simulink model "CM745A_Sci30CfgAndUse"  (R2013b)
settings: Solver=ode45  StartTime=0.0  StopTime=10.0  RelTol=1e-3
libraries: simulink x12
(part 1 of 3)
settings Model: Creator=fz41t8  LastModifiedBy=fz41t8

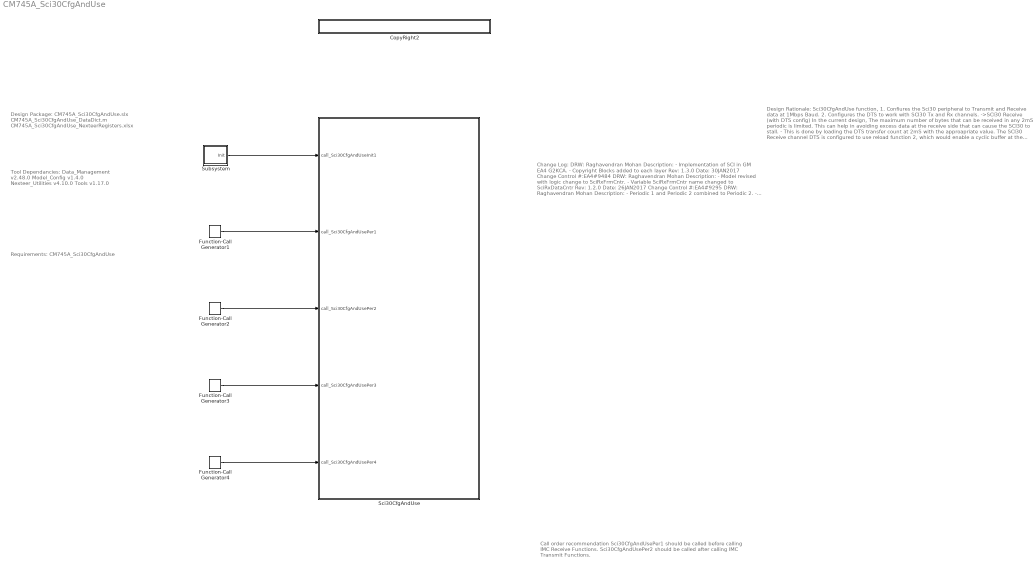
== system CM745A_Sci30CfgAndUse ==
  note: Call order recommendation
      |
      | Sci30CfgAndUsePer1 should be called before calling IMC Receive Functions.
      | Sci30CfgAndUsePer2 should be called after calling IMC Transmit Functions.
  note: Design Rationale:
      |
      | Sci30CfgAndUse function,
      | 1. Confiures the Sci30 peripheral to Transmit and Receive data at 1Mbps Baud.
      | 2. Configures the DTS to work with SCI30 Tx and Rx channels.
      |
      | ->SCI30 Receive (with DTS config)
      | In the current design, The maximum number of bytes that can be received in any
      | 2mS periodic is limited. This can help in avoiding excess data at the receive side
      | that can cause the SCI30 to stall.
      |  - This is done by loading the DTS transfer count at 2mS with the approapriate
      | value.
      | The SCI30 Receive channel DTS is configured to use reload function 2, which
      | would enable a cyclic buffer at the SCI30 receive.
      |  - This is done by configuring the address reload count. (Reload Function 2).
      |
      | ->SCI30 Transmit (with DTS config)
      | The amount of data to be sent out through the SCI30 Transmit channel is
      | loaded onto the DTS transfer count.(the number of DMA transfers equals
      | the amount of data sent out).
      | - This is done by reloading the DTS transfer count register with the actual
      |   amount of data.
      |
      | ->SCI30 Receive Channel Diagnostics
      | Sci30CfgAndUsePer2 function checks to see if the Sci receive channel has
      | received maximum amount of data and upon receiving maximum data it
      | checks for the overrun error, parity error or frame error and clears them if set.
      | This helps in preventing the SCI30 from stalling.
      |
      | Transmit - Channel master settings
      | SPID	2
      | PEID	1
      | UM		1
      |
      | Receive - Channel master settings
      | SPID	3
      | PEID	1
      | UM		1
      |
      | The DTS Channel Master settings need to be configured in SUPERVISOR Mode.
      |
      | Corruption of any of the registers would result in invalid data being sent to the other ECU.
      | And this would be the rationale behind why we dont need Protection for the SCI and DTS registers.
      | The SCI is not part of any protection, or PBG configuration.
      |
      |
      |
      | Sub-Function				rate (ms)
      |
      | Sci30CfgAndUsePer1			2			Required in all operating states
      | Sci30CfgAndUsePer2			2			Required in all operating states
      | Sci30CfgAndUsePer3			10			Required in all operating states
      | Sci30CfgAndUsePer4			100			Required in all operating states
  note: Design Package:
      |
      | CM745A_Sci30CfgAndUse.slx
      | CM745A_Sci30CfgAndUse_DataDict.m
      | CM745A_Sci30CfgAndUse_NexteerRegisters.xlsx
  note: Tool Dependancies:
      |
      | Data_Management v2.48.0
      | Model_Config v1.4.0
      | Nexteer_Utilities v4.10.0
      | Tools v1.17.0
  note: Change Log:
      |
      | DRW: Raghavendran Mohan
      | Description:
      | - Implementation of SCI in GM EA4 G2KCA.
      | - Copyright Blocks added to each layer
      |
      | Rev: 1.3.0
      | Date: 30JAN2017
      | Change Control #:EA4#9484
      | DRW: Raghavendran Mohan
      | Description:
      | - Model revised with logic change to SciRxFrmCntr.
      | - Variable SciRxFrmCntr name changed to SciRxDataCntr
      |
      | Rev: 1.2.0
      | Date: 26JAN2017
      | Change Control #:EA4#9295
      | DRW: Raghavendran Mohan
      | Description:
      | - Periodic 1 and Periodic 2 combined to Periodic 2.
      | - Periodic 5 changed to Periodic1.
      | - Name change for IMC dependent global constants.
      |
      | Rev: 1.1.0
      | Date: 11NOV2016
      | Change Control #:EA4#8302
      | DRW: Raghavendran Mohan
      | Description:
      | - Configured SCI30 to work with DTS
      | - Limited the number of messages to
      |   be received by SCI in any 2 mS
      |
      | Rev: 1.0.0
      | Date: 17OCT2016
      | Change Control #:EA4#7046
      | DRW: Raghavendran Mohan
      | Description:
      | - Initial Release
  note: Requirements:
      |
      | CM745A_Sci30CfgAndUse
  CopyRight2 : Subsystem  Description=|  mask(Copyright Information){none=on}
      | Copyright info block.                                               
      |                                                                     
      | Place copyright information at the top of every subsystem in design.
      mask prompts: none "No parameters"
      mask help: Place copyright information at the top of every subsystem in design.
      mask Display:
      | NxtrConf = 'Nexteer Confidential';
      | 
      | sys = bdroot; %handle for the current model ("system")
      | first = get_param(sys,'Created');
      | first = first(end-3:end);  %year is last four digits
      | 
      | last = get_param(sys,'LastModifiedDate');
      | if isempty(last)
      |     last = datestr(now,'yyyy');
      | else
      |     last = last(end-3:end);
      | end
      | 
      | if strcmp(first,last)
      |     fprintf('%s -- Copyright %s Nexteer',NxtrConf,first)
      | else
      |     fprintf('%s -- %s%s- %s Nexteer',NxtrConf,char(169),first,last)
      | end
  Function-Call Generator1 : simulink/Ports & Subsystems/Function-Call Generator  sample_time=0.002  numberOfIterations=1
      settings: AttributesFormatString=%<sample_time>
  Function-Call Generator2 : simulink/Ports & Subsystems/Function-Call Generator  sample_time=0.002  numberOfIterations=1
      settings: AttributesFormatString=%<sample_time>
  Function-Call Generator3 : simulink/Ports & Subsystems/Function-Call Generator  sample_time=0.01  numberOfIterations=1
      settings: AttributesFormatString=%<sample_time>
  Function-Call Generator4 : simulink/Ports & Subsystems/Function-Call Generator  sample_time=0.1  numberOfIterations=1
      settings: AttributesFormatString=%<sample_time>
  Sci30CfgAndUse : Subsystem
  Subsystem : Subsystem
  wires:
  Function-Call Generator1/1 -> Sci30CfgAndUse/2(call_Sci30CfgAndUsePer1)
  Function-Call Generator2/1 -> Sci30CfgAndUse/3(call_Sci30CfgAndUsePer2)
  Function-Call Generator3/1 -> Sci30CfgAndUse/4(call_Sci30CfgAndUsePer3)
  Function-Call Generator4/1 -> Sci30CfgAndUse/5(call_Sci30CfgAndUsePer4)
  Subsystem/1(Init) -> Sci30CfgAndUse/1(call_Sci30CfgAndUseInit1)

== system CM745A_Sci30CfgAndUse/CopyRight2 ==

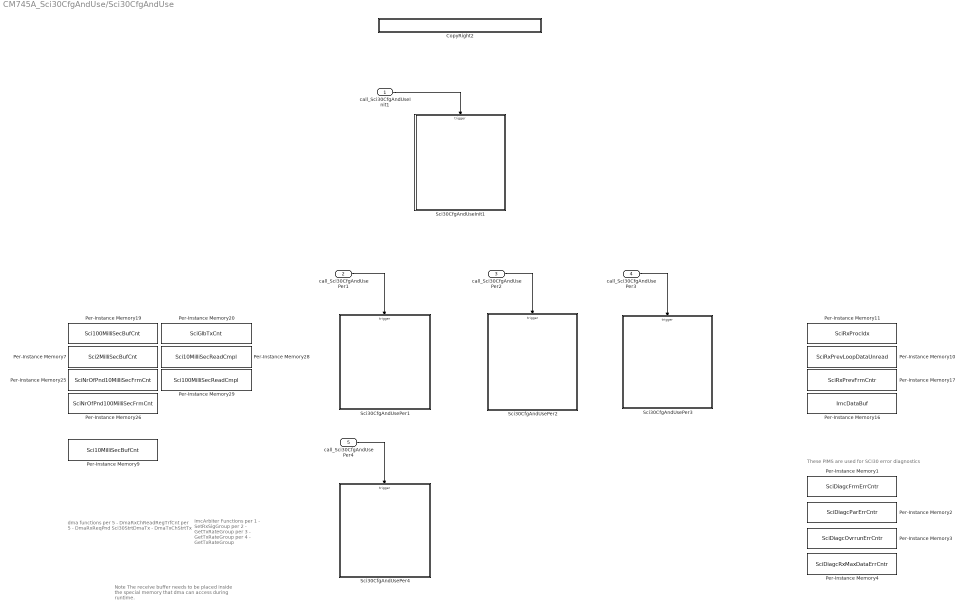
== system CM745A_Sci30CfgAndUse/Sci30CfgAndUse ==
  note: These PIMS are used for SCI30 error diagnostics
  note: Note
      |
      | The receive buffer needs to be placed
      | inside the special memory that dma can access
      |  during runtime.
  note: ImcArbiter Functions
      |
      | per 1 - SetRxSigGroup
      | per 2 - GetTxRateGroup
      | per 3 - GetTxRateGroup
      | per 4 - GetTxRateGroup
  note: dma functions
      |
      | per 5 - 				DmaRxChReadRegTrfCnt
      | per 5 - 				DmaRxReqPnd
      | Sci30StrtDmaTx - 	DmaTxChStrtTx
  call_Sci30CfgAndUseInit1 : Inport
  call_Sci30CfgAndUsePer1 : Inport  Port=2
  call_Sci30CfgAndUsePer2 : Inport  Port=3
  call_Sci30CfgAndUsePer3 : Inport  Port=4
  call_Sci30CfgAndUsePer4 : Inport  Port=5
  CopyRight2 : Subsystem  Description=|  mask(Copyright Information){none=on}
      | Copyright info block.                                               
      |                                                                     
      | Place copyright information at the top of every subsystem in design.
      mask prompts: none "No parameters"
      mask help: Place copyright information at the top of every subsystem in design.
      mask Display:
      | NxtrConf = 'Nexteer Confidential';
      | 
      | sys = bdroot; %handle for the current model ("system")
      | first = get_param(sys,'Created');
      | first = first(end-3:end);  %year is last four digits
      | 
      | last = get_param(sys,'LastModifiedDate');
      | if isempty(last)
      |     last = datestr(now,'yyyy');
      | else
      |     last = last(end-3:end);
      | end
      | 
      | if strcmp(first,last)
      |     fprintf('%s -- Copyright %s Nexteer',NxtrConf,first)
      | else
      |     fprintf('%s -- %s%s- %s Nexteer',NxtrConf,char(169),first,last)
      | end
  Per-Instance Memory1 : DataStoreMemory  RequirementInfo={} %GIDa_b3b57849_cbb3_4377_a3cb_912e17b0b2a0  DataStoreName=SciDiagcFrmErrCntr  OutDataTypeStr=uint32  StateMustResolveToSignalObject=on
  Per-Instance Memory10 : DataStoreMemory  RequirementInfo={} %GIDa_4ed7bc09_7e9a_458d_afd1_2a330d829650  DataStoreName=SciRxPrevLoopDataUnread  StateMustResolveToSignalObject=on
  Per-Instance Memory11 : DataStoreMemory  RequirementInfo={} %GIDa_3ccbf926_e816_4ba1_aa33_6f8a7244583b  DataStoreName=SciRxProcIdx  StateMustResolveToSignalObject=on
  Per-Instance Memory16 : DataStoreMemory  RequirementInfo={} %GIDa_a4699ec3_7b23_4e85_92c1_3b8b276d6679  DataStoreName=ImcDataBuf  InitialValue=[0,0,0,0,0,0,0,0]  OutDataTypeStr=uint8
  Per-Instance Memory17 : DataStoreMemory  RequirementInfo={} %GIDa_b61881d6_4c07_453b_890e_34f27dc90187  DataStoreName=SciRxPrevFrmCntr  StateMustResolveToSignalObject=on
  Per-Instance Memory19 : DataStoreMemory  RequirementInfo={} %GIDa_ab8726e9_5ac4_4e9c_b3bf_e5d79526c9cb  DataStoreName=Sci100MilliSecBufCnt  InitialValue=[]  VectorParams1D=off  StateMustResolveToSignalObject=on
  Per-Instance Memory2 : DataStoreMemory  RequirementInfo={} %GIDa_88ddc365_cba9_41ff_9af8_4f3bc4bcdd94  DataStoreName=SciDiagcParErrCntr  OutDataTypeStr=uint32  StateMustResolveToSignalObject=on
  Per-Instance Memory20 : DataStoreMemory  RequirementInfo={} %GIDa_d7519dc7_a6fd_4090_8a65_d6acf3c90b4e  DataStoreName=SciGlbTxCnt  OutDataTypeStr=uint8
  Per-Instance Memory25 : DataStoreMemory  RequirementInfo={} %GIDa_d42e51a1_a818_4595_ab2d_fbf8ed86b046  DataStoreName=SciNrOfPnd10MilliSecFrmCnt  OutDataTypeStr=uint8  StateMustResolveToSignalObject=on
  Per-Instance Memory26 : DataStoreMemory  RequirementInfo={} %GIDa_f5e07739_10f3_40b7_aa65_e2f998123e89  DataStoreName=SciNrOfPnd100MilliSecFrmCnt  OutDataTypeStr=uint8  StateMustResolveToSignalObject=on
  Per-Instance Memory28 : DataStoreMemory  RequirementInfo={} %GIDa_48b46abc_e5dd_4b66_8fa5_e2298010fa14  DataStoreName=Sci10MilliSecReadCmpl  OutDataTypeStr=boolean  StateMustResolveToSignalObject=on
  Per-Instance Memory29 : DataStoreMemory  RequirementInfo={} %GIDa_dd6879f0_97cd_4846_96b6_db1da32b280f  DataStoreName=Sci100MilliSecReadCmpl  OutDataTypeStr=boolean  StateMustResolveToSignalObject=on
  Per-Instance Memory3 : DataStoreMemory  RequirementInfo={} %GIDa_7153fc19_d7c8_405e_b0c8_79396bfd99b1  DataStoreName=SciDiagcOvrrunErrCntr  OutDataTypeStr=uint32  StateMustResolveToSignalObject=on
  Per-Instance Memory4 : DataStoreMemory  RequirementInfo={} %GIDa_3839a9f4_ebd7_4d8c_aa5f_02934402c7a8  DataStoreName=SciDiagcRxMaxDataErrCntr  OutDataTypeStr=uint32  StateMustResolveToSignalObject=on
  Per-Instance Memory7 : DataStoreMemory  RequirementInfo={} %GIDa_9668f34c_3dff_4881_9619_19e89a11e5d7  DataStoreName=Sci2MilliSecBufCnt  InitialValue=[]  OutDataTypeStr=uint8  StateMustResolveToSignalObject=on
  Per-Instance Memory9 : DataStoreMemory  RequirementInfo={} %GIDa_355f0922_cfd3_4bc4_b51e_9084d08cfe53  DataStoreName=Sci10MilliSecBufCnt  InitialValue=[]  OutDataTypeStr=uint8  StateMustResolveToSignalObject=on
  Sci30CfgAndUseInit1 : Subsystem  TreatAsAtomicUnit=on
  Sci30CfgAndUsePer1 : Subsystem  RequirementInfo={'linktype_rmi_doors' '00011b59 (/ESG Group/FDD Module Requirements/EA4 Specific/CM745A_Sci30CfgAndUse)' '#CM745A_28' 'true' 'REQ: CM745A_28' '' } %GIDa_bf038dd7_1ab4_4b18_b135_ed2bcc78b1b0  TreatAsAtomicUnit=on
  Sci30CfgAndUsePer2 : Subsystem  RequirementInfo={'linktype_rmi_doors' '00011b59 (/ESG Group/FDD Module Requirements/EA4 Specific/CM745A_Sci30CfgAndUse)' '#CM745A_25' 'true' 'REQ: CM745A_25' '' } %GIDa_256e35fd_67e5_4b63_bd20_7618d4918bb6  TreatAsAtomicUnit=on
  Sci30CfgAndUsePer3 : Subsystem  RequirementInfo={'linktype_rmi_doors' '00011b59 (/ESG Group/FDD Module Requirements/EA4 Specific/CM745A_Sci30CfgAndUse)' '#CM745A_26' 'true' 'REQ: CM745A_26' '' } %GIDa_9e620a39_8a29_406c_9071_7abfd40cb07e  TreatAsAtomicUnit=on
  Sci30CfgAndUsePer4 : Subsystem  RequirementInfo={'linktype_rmi_doors' '00011b59 (/ESG Group/FDD Module Requirements/EA4 Specific/CM745A_Sci30CfgAndUse)' '#CM745A_27' 'true' 'REQ: CM745A_27' '' } %GIDa_e30a56bb_70ac_43bc_bb33_116577e74951  TreatAsAtomicUnit=on
  wires:
  call_Sci30CfgAndUseInit1/1 -> Sci30CfgAndUseInit1/Trigger
  call_Sci30CfgAndUsePer1/1 -> Sci30CfgAndUsePer1/Trigger
  call_Sci30CfgAndUsePer2/1 -> Sci30CfgAndUsePer2/Trigger
  call_Sci30CfgAndUsePer3/1 -> Sci30CfgAndUsePer3/Trigger
  call_Sci30CfgAndUsePer4/1 -> Sci30CfgAndUsePer4/Trigger

== system CM745A_Sci30CfgAndUse/Subsystem ==
  CopyRight2 : Subsystem  Description=|  mask(Copyright Information){none=on}
      | Copyright info block.                                               
      |                                                                     
      | Place copyright information at the top of every subsystem in design.
      mask prompts: none "No parameters"
      mask help: Place copyright information at the top of every subsystem in design.
      mask Display:
      | NxtrConf = 'Nexteer Confidential';
      | 
      | sys = bdroot; %handle for the current model ("system")
      | first = get_param(sys,'Created');
      | first = first(end-3:end);  %year is last four digits
      | 
      | last = get_param(sys,'LastModifiedDate');
      | if isempty(last)
      |     last = datestr(now,'yyyy');
      | else
      |     last = last(end-3:end);
      | end
      | 
      | if strcmp(first,last)
      |     fprintf('%s -- Copyright %s Nexteer',NxtrConf,first)
      | else
      |     fprintf('%s -- %s%s- %s Nexteer',NxtrConf,char(169),first,last)
      | end
  Enabled Subsystem : Subsystem  TreatAsAtomicUnit=on
  Step : Step  Before=1  After=0  SampleTime=0
  Init : Outport
  wires:
  Enabled Subsystem/1(Init) -> Init/1
  Step/1 -> Enabled Subsystem/Enable

== system CM745A_Sci30CfgAndUse/Sci30CfgAndUse/CopyRight2 ==

== system CM745A_Sci30CfgAndUse/Sci30CfgAndUse/Sci30CfgAndUseInit1 ==
  note: This Function initializes the SCI30 Tx and Rx channels to communicate at 1Mbps Baud Rate.
      | This Function configures the DTS to work with SCI30 Tx(DTS 88) and Rx(DTS 87).
  note: DMA-DTS Register Configuration
  note: Configure SCI30 peripheral using sheet NexteerSCI30Registers inside CM745A_Sci30CfgAndUse_NexteerRegisters.xlsx
  note: Please find SCI30 DTS register configurations in SCI30CfgAndUseDTS.xlsx
      |
      | PSEUDO CODE
      |
      |
      | DTS CHANNEL 88 SCI30 TRANSMIT CONFIGURATION
      |
      | DMASSDTFSL088 = 0;
      | DMASSDTSA088 = (uint32)&SciGlbTxBuf[0];
      | DMASSDTDA088 = (uint32)&SCI30TDR;
      | DMASSDTTC088 = 0;
      | DMASSDTTCT088 = 256;
      |
      | DMASSDTFSC088 = 1;
      | DMASSDTFSL088 = 1;
      |
      |
      |
      | DTS CHANNEL 87 SCI30 RECEIVE CONFIGURATION
      |
      | DMASSDTFSL087 = 0;
      | DMASSDTSA087 = (uint32)&SCI30RDR;
      | DMASSDTDA087 = (uint32)&SciGlbRxBuf[0];
      | DMASSDTTC087 = 8388736;
      | DMASSDTTCT087 = 6208;
      |
      | DMASSDTRSA087 = (uint32)&SCI30RDR;
      | DMASSDTRDA087 = (uint32)&SciGlbRxBuf[0];
      | DMASSDTRTC087 |= 8388608;
      |
      | DMASSDTFSC087 = 1;
      | DMASSDTFSL087 = 1;
  note: Configure DMA DTS channel 87 and 88 using sheet NexteerDTSRegisters inside CM745A_Sci30CfgAndUse_NexteerRegisters.xlsx
  function : TriggerPort  TriggerType=function-call
  CopyRight2 : Subsystem  Description=|  mask(Copyright Information){none=on}
      | Copyright info block.                                               
      |                                                                     
      | Place copyright information at the top of every subsystem in design.
      mask prompts: none "No parameters"
      mask help: Place copyright information at the top of every subsystem in design.
      mask Display:
      | NxtrConf = 'Nexteer Confidential';
      | 
      | sys = bdroot; %handle for the current model ("system")
      | first = get_param(sys,'Created');
      | first = first(end-3:end);  %year is last four digits
      | 
      | last = get_param(sys,'LastModifiedDate');
      | if isempty(last)
      |     last = datestr(now,'yyyy');
      | else
      |     last = last(end-3:end);
      | end
      | 
      | if strcmp(first,last)
      |     fprintf('%s -- Copyright %s Nexteer',NxtrConf,first)
      | else
      |     fprintf('%s -- %s%s- %s Nexteer',NxtrConf,char(169),first,last)
      | end

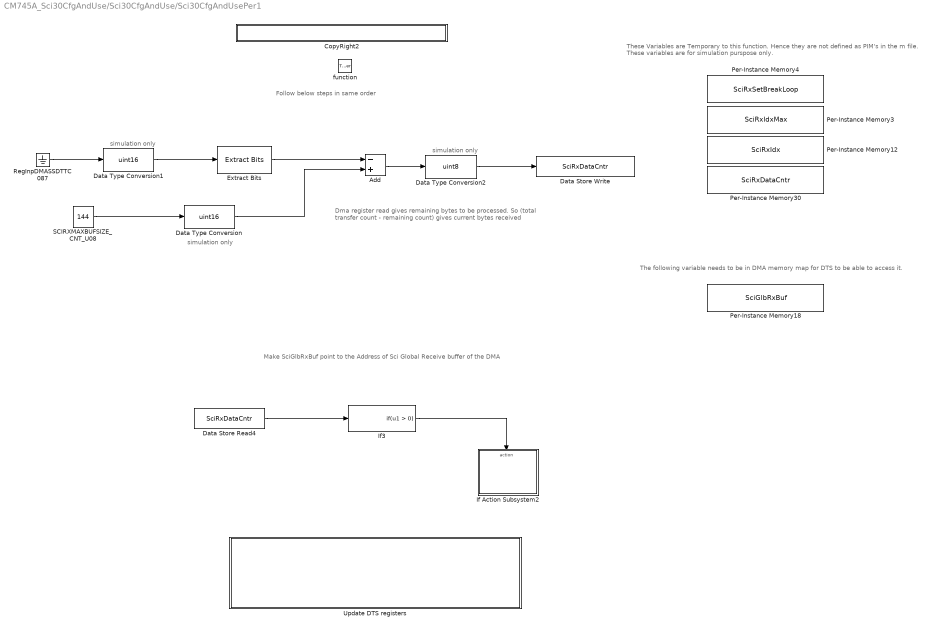
== system CM745A_Sci30CfgAndUse/Sci30CfgAndUse/Sci30CfgAndUsePer1 ==
  note: simulation only
  note: Dma register read gives remaining bytes to be processed.
      | So (total transfer count - remaining count) gives current bytes received
  note: Make SciGlbRxBuf point to the Address of Sci Global Receive buffer of the DMA
  note: Follow below steps in same order
  note: These Variables are Temporary to this function. Hence they are not defined as PIM's in the m file.
      | These variables are for simulation purspose only.
  note: simulation only
  note: simulation only
  note: The following variable needs to be in DMA memory map for DTS to be able to access it.
  function : TriggerPort  TriggerType=function-call
  Add : Sum  Inputs=-+
  CopyRight2 : Subsystem  Description=|  mask(Copyright Information){none=on}
      | Copyright info block.                                               
      |                                                                     
      | Place copyright information at the top of every subsystem in design.
      mask prompts: none "No parameters"
      mask help: Place copyright information at the top of every subsystem in design.
      mask Display:
      | NxtrConf = 'Nexteer Confidential';
      | 
      | sys = bdroot; %handle for the current model ("system")
      | first = get_param(sys,'Created');
      | first = first(end-3:end);  %year is last four digits
      | 
      | last = get_param(sys,'LastModifiedDate');
      | if isempty(last)
      |     last = datestr(now,'yyyy');
      | else
      |     last = last(end-3:end);
      | end
      | 
      | if strcmp(first,last)
      |     fprintf('%s -- Copyright %s Nexteer',NxtrConf,first)
      | else
      |     fprintf('%s -- %s%s- %s Nexteer',NxtrConf,char(169),first,last)
      | end
  Data Store Read4 : DataStoreRead  DataStoreName=SciRxDataCntr
  Data Store Write : DataStoreWrite  DataStoreName=SciRxDataCntr
  Data Type Conversion : DataTypeConversion  OutDataTypeStr=uint16
  Data Type Conversion1 : DataTypeConversion  OutDataTypeStr=uint16
  Data Type Conversion2 : DataTypeConversion  OutDataTypeStr=uint8
  Extract Bits : simulink/Logic and Bit Operations/Extract Bits  bitsToExtract=Range of bits  numBits=8  bitIdxRange=[0 15]  outScalingMode=Preserve fixed-point scaling
  If Action Subsystem2 : Subsystem  TreatAsAtomicUnit=on
  If3 : If  ShowElse=off
      settings: AttributesFormatString=%<IfExpression>
  Per-Instance Memory12 : DataStoreMemory  RequirementInfo={} %GIDa_10aec818_c7eb_44be_9468_3f861d56c791  DataStoreName=SciRxIdx  OutDataTypeStr=uint8
  Per-Instance Memory18 : DataStoreMemory  RequirementInfo={} %GIDa_9eb3493f_f4d3_4ae6_8599_8ce3936fda0e  DataStoreName=SciGlbRxBuf  InitialValue=[0,0,0,0,0,0,0,0]  OutDataTypeStr=uint8
  Per-Instance Memory3 : DataStoreMemory  RequirementInfo={} %GIDa_0f1d5dec_99dd_48b3_81e2_7cc92f58afeb  DataStoreName=SciRxIdxMax  OutDataTypeStr=uint8
  Per-Instance Memory30 : DataStoreMemory  RequirementInfo={} %GIDa_67fcd88a_9e09_4a74_a9c0_611da1fab4fa  DataStoreName=SciRxDataCntr
  Per-Instance Memory4 : DataStoreMemory  RequirementInfo={} %GIDa_846dd6da_f32a_4fb1_951f_9840ad07db99  DataStoreName=SciRxSetBreakLoop  OutDataTypeStr=boolean
  RegInpDMASSDTTC087 : Ground
  SCIRXMAXBUFSIZE_CNT_U08 : Constant  Value=144  OutDataTypeStr=uint8
  Update DTS registers : Subsystem
  wires:
  Data Store Read4/1 -> If3/1
  If3/1 -> If Action Subsystem2/Action
  Extract Bits/1 -> Add/1
  Data Type Conversion1/1 -> Extract Bits/1
  RegInpDMASSDTTC087/1 -> Data Type Conversion1/1
  SCIRXMAXBUFSIZE_CNT_U08/1 -> Data Type Conversion/1
  Data Type Conversion/1 -> Add/2
  Data Type Conversion2/1 -> Data Store Write/1
  Add/1 -> Data Type Conversion2/1

== system CM745A_Sci30CfgAndUse/Sci30CfgAndUse/Sci30CfgAndUsePer2 ==
  note: This Data needs to be put in exclusive
      | memory, that has read/write protection.
      | (To prevent Read Write Collision)
  note: Conditional Compile (Based on IMC Arbitration of 2 Millisec Rate Group !=0)
  note: Follow below steps in same order
  note: This Data needs to be put in exclusive
      | memory, that has read/write protection.
      | (To prevent Read Write Collision)
  function : TriggerPort  TriggerType=function-call
  CopyRight2 : Subsystem  Description=|  mask(Copyright Information){none=on}
      | Copyright info block.                                               
      |                                                                     
      | Place copyright information at the top of every subsystem in design.
      mask prompts: none "No parameters"
      mask help: Place copyright information at the top of every subsystem in design.
      mask Display:
      | NxtrConf = 'Nexteer Confidential';
      | 
      | sys = bdroot; %handle for the current model ("system")
      | first = get_param(sys,'Created');
      | first = first(end-3:end);  %year is last four digits
      | 
      | last = get_param(sys,'LastModifiedDate');
      | if isempty(last)
      |     last = datestr(now,'yyyy');
      | else
      |     last = last(end-3:end);
      | end
      | 
      | if strcmp(first,last)
      |     fprintf('%s -- Copyright %s Nexteer',NxtrConf,first)
      | else
      |     fprintf('%s -- %s%s- %s Nexteer',NxtrConf,char(169),first,last)
      | end
  Data Store Read1 : DataStoreRead  DataStoreName=Sci2MilliSecBufCnt
  Data Store Write1 : DataStoreWrite  DataStoreName=Sci2MilliSecReadCmpl
  GetTxRateGroup : Subsystem
  IMCARBN_NROF2MILLISECRATEGROUP_CNT_U08 : Constant  Value=0  OutDataTypeStr=uint8
  IMCARBN_RATEGROUPID2MILLISEC_CNT_U08 : Constant  Value=0  OutDataTypeStr=uint8
  Per-Instance Memory27 : DataStoreMemory  RequirementInfo={} %GIDa_fa2153ee_75ad_4194_bafc_e32e8d6d4301  DataStoreName=Sci2MilliSecReadCmpl  OutDataTypeStr=boolean
  Sci30Transmit : Subsystem  RequirementInfo={'linktype_rmi_doors' '00011b59 (/ESG Group/FDD Module Requirements/EA4 Specific/CM745A_Sci30CfgAndUse)' '#CM745A_24' 'true' 'REQ: CM745A_24' '' } %GIDa_898b519a_4f36_4d71_a508_ee16e2031590  TreatAsAtomicUnit=on
  Terminator : Terminator
  wires:
  IMCARBN_NROF2MILLISECRATEGROUP_CNT_U08/1 -> Terminator/1
  GetTxRateGroup/1(Sci2MilliSecReadCmplCnt) -> Data Store Write1/1
  Data Store Read1/1 -> GetTxRateGroup/2(Sci2MilliSecBufCnt)
  IMCARBN_RATEGROUPID2MILLISEC_CNT_U08/1 -> GetTxRateGroup/1(IMCARBN_RATEGROUPID2MILLISEC)

== system CM745A_Sci30CfgAndUse/Sci30CfgAndUse/Sci30CfgAndUsePer3 ==
  note: Conditional Compile (Based on IMC Arbitration of 2 Millisec Rate Group !=0)
  note: Follow below steps in same order
  note: This Data needs to be put in exclusive
      | memory, that has read/write protection.
      | (To prevent Read Write Collision)
  note: This Data needs to be put in exclusive
      | memory, that has read/write protection.
      | (To prevent Read Write Collision)
  note: This Data needs to be put in exclusive
      | memory, that has read/write protection.
      | (To prevent Read Write Collision)
  function : TriggerPort  TriggerType=function-call
  CopyRight2 : Subsystem  Description=|  mask(Copyright Information){none=on}
      | Copyright info block.                                               
      |                                                                     
      | Place copyright information at the top of every subsystem in design.
      mask prompts: none "No parameters"
      mask help: Place copyright information at the top of every subsystem in design.
      mask Display:
      | NxtrConf = 'Nexteer Confidential';
      | 
      | sys = bdroot; %handle for the current model ("system")
      | first = get_param(sys,'Created');
      | first = first(end-3:end);  %year is last four digits
      | 
      | last = get_param(sys,'LastModifiedDate');
      | if isempty(last)
      |     last = datestr(now,'yyyy');
      | else
      |     last = last(end-3:end);
      | end
      | 
      | if strcmp(first,last)
      |     fprintf('%s -- Copyright %s Nexteer',NxtrConf,first)
      | else
      |     fprintf('%s -- %s%s- %s Nexteer',NxtrConf,char(169),first,last)
      | end
  Data Store Read1 : DataStoreRead  DataStoreName=Sci10MilliSecBufCnt
  Data Store Write : DataStoreWrite  DataStoreName=SciNrOfPnd10MilliSecFrmCnt
  Data Store Write1 : DataStoreWrite  DataStoreName=Sci10MilliSecReadCmpl
  GetTxRateGroup : Subsystem
  IMCARBN_NROF10MILLISECRATEGROUP_CNT_U08 : Constant  Value=0  OutDataTypeStr=uint8
  IMCARBN_RATEGROUPID10MILLISEC_CNT_U08 : Constant  Value=0  OutDataTypeStr=uint8
  wires:
  IMCARBN_NROF10MILLISECRATEGROUP_CNT_U08/1 -> Data Store Write/1
  GetTxRateGroup/1(Sci10MilliSecReadCmplCnt) -> Data Store Write1/1
  Data Store Read1/1 -> GetTxRateGroup/2(Sci10MilliSecBufCnt)
  IMCARBN_RATEGROUPID10MILLISEC_CNT_U08/1 -> GetTxRateGroup/1(IMCARBN_RATEGROUPID10MILLISEC)

== system CM745A_Sci30CfgAndUse/Sci30CfgAndUse/Sci30CfgAndUsePer4 ==
  note: Follow below steps in same order
  note: Conditional Compile (Based on IMC Arbitration of 2 Millisec Rate Group !=0)
  note: This Data needs to be put in exclusive
      | memory, that has read/write protection.
      | (To prevent Read Write Collision)
  note: This Data needs to be put in exclusive
      | memory, that has read/write protection.
      | (To prevent Read Write Collision)
  note: This Data needs to be put in exclusive
      | memory, that has read/write protection.
      | (To prevent Read Write Collision)
  function : TriggerPort  TriggerType=function-call
  CopyRight2 : Subsystem  Description=|  mask(Copyright Information){none=on}
      | Copyright info block.                                               
      |                                                                     
      | Place copyright information at the top of every subsystem in design.
      mask prompts: none "No parameters"
      mask help: Place copyright information at the top of every subsystem in design.
      mask Display:
      | NxtrConf = 'Nexteer Confidential';
      | 
      | sys = bdroot; %handle for the current model ("system")
      | first = get_param(sys,'Created');
      | first = first(end-3:end);  %year is last four digits
      | 
      | last = get_param(sys,'LastModifiedDate');
      | if isempty(last)
      |     last = datestr(now,'yyyy');
      | else
      |     last = last(end-3:end);
      | end
      | 
      | if strcmp(first,last)
      |     fprintf('%s -- Copyright %s Nexteer',NxtrConf,first)
      | else
      |     fprintf('%s -- %s%s- %s Nexteer',NxtrConf,char(169),first,last)
      | end
  Data Store Read1 : DataStoreRead  DataStoreName=Sci100MilliSecBufCnt
  Data Store Write : DataStoreWrite  DataStoreName=SciNrOfPnd100MilliSecFrmCnt
  Data Store Write1 : DataStoreWrite  DataStoreName=Sci100MilliSecReadCmpl
  GetTxRateGroup : Subsystem
  IMCARBN_NROF100MILLISECRATEGROUP_CNT_U08 : Constant  OutDataTypeStr=uint8
  IMCARBN_RATEGROUPID100MILLISEC_CNT_U08 : Constant  OutDataTypeStr=uint8
  wires:
  IMCARBN_NROF100MILLISECRATEGROUP_CNT_U08/1 -> Data Store Write/1
  GetTxRateGroup/1(Sci100MilliSecReadCmplCnt) -> Data Store Write1/1
  Data Store Read1/1 -> GetTxRateGroup/2(Sci100MilliSecBufCnt)
  IMCARBN_RATEGROUPID100MILLISEC_CNT_U08/1 -> GetTxRateGroup/1(IMCARBN_RATEGROUPID100MILLISEC)

== system CM745A_Sci30CfgAndUse/Subsystem/CopyRight2 ==

== system CM745A_Sci30CfgAndUse/Subsystem/Enabled Subsystem ==
  Enable : EnablePort
  CopyRight2 : Subsystem  Description=|  mask(Copyright Information){none=on}
      | Copyright info block.                                               
      |                                                                     
      | Place copyright information at the top of every subsystem in design.
      mask prompts: none "No parameters"
      mask help: Place copyright information at the top of every subsystem in design.
      mask Display:
      | NxtrConf = 'Nexteer Confidential';
      | 
      | sys = bdroot; %handle for the current model ("system")
      | first = get_param(sys,'Created');
      | first = first(end-3:end);  %year is last four digits
      | 
      | last = get_param(sys,'LastModifiedDate');
      | if isempty(last)
      |     last = datestr(now,'yyyy');
      | else
      |     last = last(end-3:end);
      | end
      | 
      | if strcmp(first,last)
      |     fprintf('%s -- Copyright %s Nexteer',NxtrConf,first)
      | else
      |     fprintf('%s -- %s%s- %s Nexteer',NxtrConf,char(169),first,last)
      | end
  Function Call Trigger : simulink/Ports & Subsystems/Function-Call Generator  RequirementInfo="{'linktype_rmi_doors' '000089e3 (/E-STEER_New/System Specification Documents/Core Specs/Subsystem Specs/System Functions FDD/SF-46  Gross Cross Check)' '#211' 'true' 'REQ: SF046A_211' '' ; 'linktype_rmi_doors' '000089e3 (/E-STEER_New/System Specification Documents/Core Specs/Subsystem Specs/System Functions FDD/SF-46  Gross Cross Check)' '#182' 'true' 'REQ: SF046A_182' '' } %GIDa_cf5bacff_48a9_4312_b446_700ab36e3d94"  sample_time=0.002  numberOfIterations=1
      settings: AttributesFormatString=%<sample_time>
  Init : Outport
  wires:
  Function Call Trigger/1 -> Init/1

== system CM745A_Sci30CfgAndUse/Sci30CfgAndUse/Sci30CfgAndUseInit1/CopyRight2 ==

== system CM745A_Sci30CfgAndUse/Sci30CfgAndUse/Sci30CfgAndUsePer1/CopyRight2 ==

== system CM745A_Sci30CfgAndUse/Sci30CfgAndUse/Sci30CfgAndUsePer1/If Action Subsystem2 ==
  note: Follow below steps in same order
  Action Port : ActionPort  ActionType=then
  Add : Sum
  Constant : Constant  Value=0  OutDataTypeStr=boolean
  Constant1 : Constant  Value=0  OutDataTypeStr=uint8
  Constant2 : Constant  Value=0  OutDataTypeStr=uint8
  CopyRight2 : Subsystem  Description=|  mask(Copyright Information){none=on}
      | Copyright info block.                                               
      |                                                                     
      | Place copyright information at the top of every subsystem in design.
      mask prompts: none "No parameters"
      mask help: Place copyright information at the top of every subsystem in design.
      mask Display:
      | NxtrConf = 'Nexteer Confidential';
      | 
      | sys = bdroot; %handle for the current model ("system")
      | first = get_param(sys,'Created');
      | first = first(end-3:end);  %year is last four digits
      | 
      | last = get_param(sys,'LastModifiedDate');
      | if isempty(last)
      |     last = datestr(now,'yyyy');
      | else
      |     last = last(end-3:end);
      | end
      | 
      | if strcmp(first,last)
      |     fprintf('%s -- Copyright %s Nexteer',NxtrConf,first)
      | else
      |     fprintf('%s -- %s%s- %s Nexteer',NxtrConf,char(169),first,last)
      | end
  Data Store Read1 : DataStoreRead  DataStoreName=SciRxDataCntr
  Data Store Read3 : DataStoreRead  DataStoreName=SciRxPrevLoopDataUnread
  Data Store Read4 : DataStoreRead  DataStoreName=SciRxDataCntr
  Data Store Write : DataStoreWrite  DataStoreName=SciRxIdx
  Data Store Write1 : DataStoreWrite  DataStoreName=SciRxPrevLoopDataUnread
  Data Store Write2 : DataStoreWrite  DataStoreName=SciRxIdxMax
  Data Store Write3 : DataStoreWrite  DataStoreName=SciRxPrevFrmCntr
  While Iterator Subsystem : Subsystem  RequirementInfo={'linktype_rmi_doors' '00011b59 (/ESG Group/FDD Module Requirements/EA4 Specific/CM745A_Sci30CfgAndUse)' '#CM745A_35' 'true' 'REQ: CM745A_35' '' } %GIDa_a7febead_a2f3_48b5_a7e9_dbc4923b1949  TreatAsAtomicUnit=on
  wires:
  Constant/1 -> While Iterator Subsystem/1(IC)
  Data Store Read1/1 -> Data Store Write3/1
  Constant1/1 -> Data Store Write/1
  Constant2/1 -> Data Store Write1/1
  Data Store Read3/1 -> Add/2
  Add/1 -> Data Store Write2/1
  Data Store Read4/1 -> Add/1

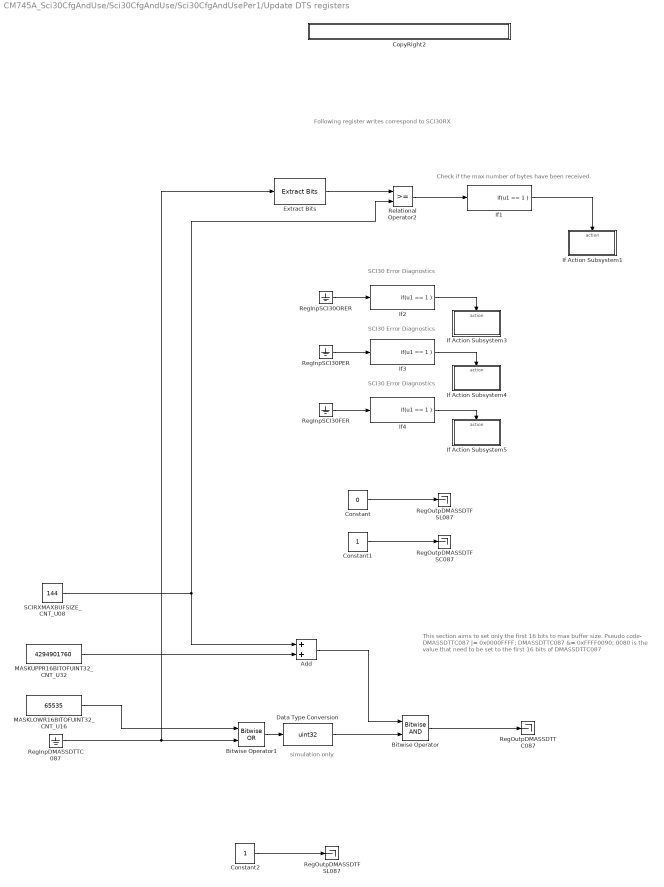
== system CM745A_Sci30CfgAndUse/Sci30CfgAndUse/Sci30CfgAndUsePer1/Update DTS registers ==
  note: Check if the max number of bytes have been received.
  note: This section aims to set only the first 16 bits to max buffer size.
      | Pseudo code-
      |
      | DMASSDTTC087 |= 0x0000FFFF;
      | DMASSDTTC087 &= 0xFFFF0090;
      |
      | 0080 is the value that need to be set to the first 16 bits of DMASSDTTC087
  note: Following register writes correspond to SCI30RX
  note: simulation only
  note: SCI30 Error Diagnostics
  note: SCI30 Error Diagnostics
  note: SCI30 Error Diagnostics
  Add : Sum
  Bitwise Operator : simulink/Logic and Bit Operations/Bitwise Operator  logicop=AND  UseBitMask=off  NumInputPorts=2  BitMask=bin2dec('11011001')  BitMaskRealWorld=Stored Integer
  Bitwise Operator1 : simulink/Logic and Bit Operations/Bitwise Operator  logicop=OR  UseBitMask=off  NumInputPorts=2  BitMask=bin2dec('11011001')  BitMaskRealWorld=Stored Integer
  Constant : Constant  Value=0  OutDataTypeStr=uint8
  Constant1 : Constant  OutDataTypeStr=uint8
  Constant2 : Constant
  CopyRight2 : Subsystem  Description=|  mask(Copyright Information){none=on}
      | Copyright info block.                                               
      |                                                                     
      | Place copyright information at the top of every subsystem in design.
      mask prompts: none "No parameters"
      mask help: Place copyright information at the top of every subsystem in design.
      mask Display:
      | NxtrConf = 'Nexteer Confidential';
      | 
      | sys = bdroot; %handle for the current model ("system")
      | first = get_param(sys,'Created');
      | first = first(end-3:end);  %year is last four digits
      | 
      | last = get_param(sys,'LastModifiedDate');
      | if isempty(last)
      |     last = datestr(now,'yyyy');
      | else
      |     last = last(end-3:end);
      | end
      | 
      | if strcmp(first,last)
      |     fprintf('%s -- Copyright %s Nexteer',NxtrConf,first)
      | else
      |     fprintf('%s -- %s%s- %s Nexteer',NxtrConf,char(169),first,last)
      | end
  Data Type Conversion : DataTypeConversion  OutDataTypeStr=uint32
  Extract Bits : simulink/Logic and Bit Operations/Extract Bits  bitsToExtract=Range of bits  numBits=8  bitIdxRange=[0 15]  outScalingMode=Preserve fixed-point scaling
  If Action Subsystem1 : Subsystem  RequirementInfo={'linktype_rmi_doors' '00011b59 (/ESG Group/FDD Module Requirements/EA4 Specific/CM745A_Sci30CfgAndUse)' '#CM745A_39' 'true' 'REQ: CM745A_39' '' } %GIDa_f123752a_717b_4091_9fc8_a8616983ad1f  TreatAsAtomicUnit=on
  If Action Subsystem3 : Subsystem  TreatAsAtomicUnit=on
  If Action Subsystem4 : Subsystem  TreatAsAtomicUnit=on
  If Action Subsystem5 : Subsystem  TreatAsAtomicUnit=on
  If{1..4} (4 alike) : If  IfExpression=u1 == 1  ShowElse=off
  MASKLOWR16BITOFUINT32_CNT_U16 : Constant  Value=65535  OutDataTypeStr=uint16
  MASKUPPR16BITOFUINT32_CNT_U32 : Constant  Value=4294901760  OutDataTypeStr=uint32
  RegInpDMASSDTTC087 : Ground
  RegInpSCI30FER : Ground
  RegInpSCI30ORER : Ground
  RegInpSCI30PER : Ground
  RegOutpDMASSDTFSC087 : Terminator
  RegOutpDMASSDTFSL087 : Terminator
  "RegOutpDMASSDTFSL087 " : Terminator
  RegOutpDMASSDTTC087 : Terminator
  Relational Operator2 : RelationalOperator  OutDataTypeStr=boolean
  SCIRXMAXBUFSIZE_CNT_U08 : Constant  Value=144  OutDataTypeStr=uint8
  wires:
  Constant/1 -> RegOutpDMASSDTFSL087/1
  Constant1/1 -> RegOutpDMASSDTFSC087/1
  Constant2/1 -> "RegOutpDMASSDTFSL087 "/1
  RegInpDMASSDTTC087/1 -> Bitwise Operator1/2, Extract Bits/1
  SCIRXMAXBUFSIZE_CNT_U08/1 -> Relational Operator2/2, Add/1
  Extract Bits/1 -> Relational Operator2/1
  Relational Operator2/1 -> If1/1
  If1/1 -> If Action Subsystem1/Action
  MASKLOWR16BITOFUINT32_CNT_U16/1 -> Bitwise Operator1/1
  Bitwise Operator/1 -> RegOutpDMASSDTTC087/1
  Add/1 -> Bitwise Operator/1
  MASKUPPR16BITOFUINT32_CNT_U32/1 -> Add/2
  Bitwise Operator1/1 -> Data Type Conversion/1
  Data Type Conversion/1 -> Bitwise Operator/2
  RegInpSCI30ORER/1 -> If2/1
  If2/1 -> If Action Subsystem3/Action
  RegInpSCI30PER/1 -> If3/1
  If3/1 -> If Action Subsystem4/Action
  RegInpSCI30FER/1 -> If4/1
  If4/1 -> If Action Subsystem5/Action

== system CM745A_Sci30CfgAndUse/Sci30CfgAndUse/Sci30CfgAndUsePer2/CopyRight2 ==

== system CM745A_Sci30CfgAndUse/Sci30CfgAndUse/Sci30CfgAndUsePer2/GetTxRateGroup ==
  IMCARBN_RATEGROUPID2MILLISEC : Inport
  Sci2MilliSecBufCnt : Inport  Port=2
  CopyRight2 : Subsystem  Description=|  mask(Copyright Information){none=on}
      | Copyright info block.                                               
      |                                                                     
      | Place copyright information at the top of every subsystem in design.
      mask prompts: none "No parameters"
      mask help: Place copyright information at the top of every subsystem in design.
      mask Display:
      | NxtrConf = 'Nexteer Confidential';
      | 
      | sys = bdroot; %handle for the current model ("system")
      | first = get_param(sys,'Created');
      | first = first(end-3:end);  %year is last four digits
      | 
      | last = get_param(sys,'LastModifiedDate');
      | if isempty(last)
      |     last = datestr(now,'yyyy');
      | else
      |     last = last(end-3:end);
      | end
      | 
      | if strcmp(first,last)
      |     fprintf('%s -- Copyright %s Nexteer',NxtrConf,first)
      | else
      |     fprintf('%s -- %s%s- %s Nexteer',NxtrConf,char(169),first,last)
      | end
  Ground : Ground
  Terminator : Terminator
  Terminator1 : Terminator
  Sci2MilliSecReadCmplCnt : Outport
  wires:
  IMCARBN_RATEGROUPID2MILLISEC/1 -> Terminator/1
  Sci2MilliSecBufCnt/1 -> Terminator1/1
  Ground/1 -> Sci2MilliSecReadCmplCnt/1

== system CM745A_Sci30CfgAndUse/Sci30CfgAndUse/Sci30CfgAndUsePer2/Sci30Transmit ==
  note: These Variables are Temporary to this function. Hence they are not defined as PIM's in the m file.
      | These variables are for simulation purspose only.
  note: Make SciGlbTxBuf point to the Address of Sci Global Transmit buffer of the DMA
  note: Follow below steps in same order
  note: The following variable needs to be in DMA memory map for DTS to be able to access it.
  Constant1 : Constant  Value=0  OutDataTypeStr=uint8
  CopyRight2 : Subsystem  Description=|  mask(Copyright Information){none=on}
      | Copyright info block.                                               
      |                                                                     
      | Place copyright information at the top of every subsystem in design.
      mask prompts: none "No parameters"
      mask help: Place copyright information at the top of every subsystem in design.
      mask Display:
      | NxtrConf = 'Nexteer Confidential';
      | 
      | sys = bdroot; %handle for the current model ("system")
      | first = get_param(sys,'Created');
      | first = first(end-3:end);  %year is last four digits
      | 
      | last = get_param(sys,'LastModifiedDate');
      | if isempty(last)
      |     last = datestr(now,'yyyy');
      | else
      |     last = last(end-3:end);
      | end
      | 
      | if strcmp(first,last)
      |     fprintf('%s -- Copyright %s Nexteer',NxtrConf,first)
      | else
      |     fprintf('%s -- %s%s- %s Nexteer',NxtrConf,char(169),first,last)
      | end
  Data Store Read1 : DataStoreRead  DataStoreName=Sci2MilliSecReadCmpl
  Data Store Read2 : DataStoreRead  DataStoreName=Sci10MilliSecReadCmpl
  Data Store Read3 : DataStoreRead  DataStoreName=Sci100MilliSecReadCmpl
  Data Store Write : DataStoreWrite  DataStoreName=SciTxByteUsedCnt
  If : If  IfExpression=u1 == 1  ShowElse=off
      settings: AttributesFormatString=%<IfExpression>
  If Action Subsystem : Subsystem  TreatAsAtomicUnit=on
  If Action Subsystem1 : Subsystem  TreatAsAtomicUnit=on
  If Action Subsystem2 : Subsystem  TreatAsAtomicUnit=on
  If1 : If  IfExpression=u1 == 1  ShowElse=off
      settings: AttributesFormatString=%<IfExpression>
  If2 : If  IfExpression=u1 == 1  ShowElse=off
      settings: AttributesFormatString=%<IfExpression>
  Per-Instance Memory2 : DataStoreMemory  RequirementInfo={} %GIDa_e64cf529_f3ac_467c_84ab_498f6d2218ac  DataStoreName=SciTxByteUsedCnt  OutDataTypeStr=uint8
  Per-Instance Memory23 : DataStoreMemory  RequirementInfo={} %GIDa_a8e15efc_445b_42d6_a473_1bc6dc138029  DataStoreName=SciTxEmptyFrmCnt  OutDataTypeStr=uint8
  Per-Instance Memory24 : DataStoreMemory  RequirementInfo={} %GIDa_906079d6_af69_4c41_a22f_9b3ca0f7163b  DataStoreName=SciTxSigByteCnt  OutDataTypeStr=uint8
  Per-Instance Memory6 : DataStoreMemory  RequirementInfo={} %GIDa_6da2783e_aa73_4ac5_9aa7_2be4f558c163  DataStoreName=SciTxSigGroupCnt  OutDataTypeStr=uint8
  Per-Instance Memory8 : DataStoreMemory  RequirementInfo={} %GIDa_e33e0430_76a2_4ad0_a097_2173af3c9260  DataStoreName=SciGlbTxBuf  OutDataTypeStr=uint8
  Update DTS registers : Subsystem
  wires:
  If/1 -> If Action Subsystem/Action
  Data Store Read1/1 -> If/1
  If1/1 -> If Action Subsystem1/Action
  Data Store Read2/1 -> If1/1
  If2/1 -> If Action Subsystem2/Action
  Data Store Read3/1 -> If2/1
  Constant1/1 -> Data Store Write/1

== system CM745A_Sci30CfgAndUse/Sci30CfgAndUse/Sci30CfgAndUsePer3/CopyRight2 ==

== system CM745A_Sci30CfgAndUse/Sci30CfgAndUse/Sci30CfgAndUsePer3/GetTxRateGroup ==
  IMCARBN_RATEGROUPID10MILLISEC : Inport
  Sci10MilliSecBufCnt : Inport  Port=2
  CopyRight2 : Subsystem  Description=|  mask(Copyright Information){none=on}
      | Copyright info block.                                               
      |                                                                     
      | Place copyright information at the top of every subsystem in design.
      mask prompts: none "No parameters"
      mask help: Place copyright information at the top of every subsystem in design.
      mask Display:
      | NxtrConf = 'Nexteer Confidential';
      | 
      | sys = bdroot; %handle for the current model ("system")
      | first = get_param(sys,'Created');
      | first = first(end-3:end);  %year is last four digits
      | 
      | last = get_param(sys,'LastModifiedDate');
      | if isempty(last)
      |     last = datestr(now,'yyyy');
      | else
      |     last = last(end-3:end);
      | end
      | 
      | if strcmp(first,last)
      |     fprintf('%s -- Copyright %s Nexteer',NxtrConf,first)
      | else
      |     fprintf('%s -- %s%s- %s Nexteer',NxtrConf,char(169),first,last)
      | end
  Ground : Ground
  Terminator : Terminator
  Terminator1 : Terminator
  Sci10MilliSecReadCmplCnt : Outport
  wires:
  IMCARBN_RATEGROUPID10MILLISEC/1 -> Terminator/1
  Sci10MilliSecBufCnt/1 -> Terminator1/1
  Ground/1 -> Sci10MilliSecReadCmplCnt/1

== system CM745A_Sci30CfgAndUse/Sci30CfgAndUse/Sci30CfgAndUsePer4/CopyRight2 ==

== system CM745A_Sci30CfgAndUse/Sci30CfgAndUse/Sci30CfgAndUsePer4/GetTxRateGroup ==
  IMCARBN_RATEGROUPID100MILLISEC : Inport
  Sci100MilliSecBufCnt : Inport  Port=2
  CopyRight2 : Subsystem  Description=|  mask(Copyright Information){none=on}
      | Copyright info block.                                               
      |                                                                     
      | Place copyright information at the top of every subsystem in design.
      mask prompts: none "No parameters"
      mask help: Place copyright information at the top of every subsystem in design.
      mask Display:
      | NxtrConf = 'Nexteer Confidential';
      | 
      | sys = bdroot; %handle for the current model ("system")
      | first = get_param(sys,'Created');
      | first = first(end-3:end);  %year is last four digits
      | 
      | last = get_param(sys,'LastModifiedDate');
      | if isempty(last)
      |     last = datestr(now,'yyyy');
      | else
      |     last = last(end-3:end);
      | end
      | 
      | if strcmp(first,last)
      |     fprintf('%s -- Copyright %s Nexteer',NxtrConf,first)
      | else
      |     fprintf('%s -- %s%s- %s Nexteer',NxtrConf,char(169),first,last)
      | end
  Ground : Ground
  Terminator : Terminator
  Terminator1 : Terminator
  Sci100MilliSecReadCmplCnt : Outport
  wires:
  IMCARBN_RATEGROUPID100MILLISEC/1 -> Terminator/1
  Sci100MilliSecBufCnt/1 -> Terminator1/1
  Ground/1 -> Sci100MilliSecReadCmplCnt/1

== system CM745A_Sci30CfgAndUse/Subsystem/Enabled Subsystem/CopyRight2 ==

== system CM745A_Sci30CfgAndUse/Sci30CfgAndUse/Sci30CfgAndUsePer1/If Action Subsystem2/CopyRight2 ==

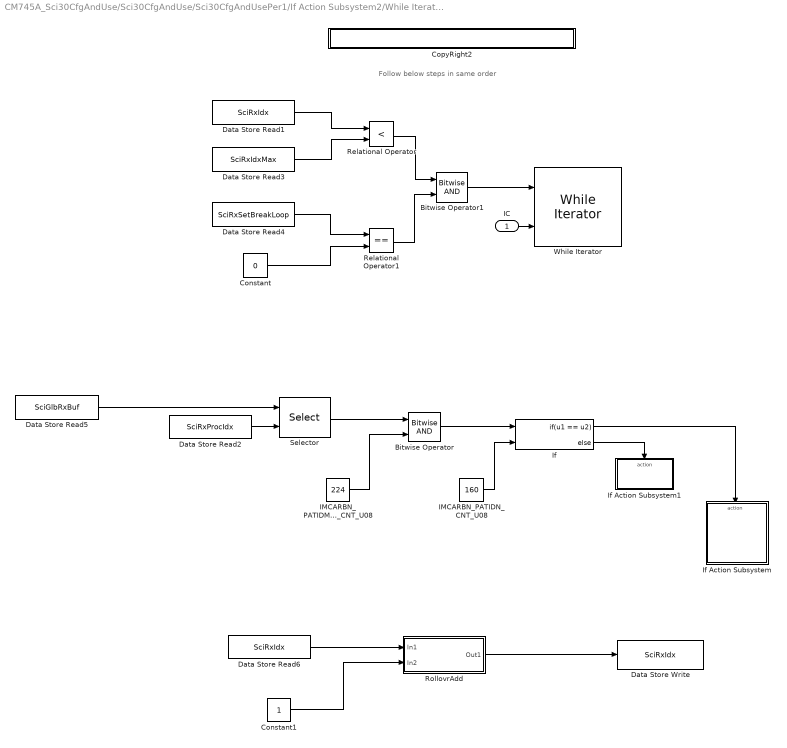
== system CM745A_Sci30CfgAndUse/Sci30CfgAndUse/Sci30CfgAndUsePer1/If Action Subsystem2/While Iterator Subsystem ==
  note: Follow below steps in same order
  IC : Inport
  Bitwise Operator : simulink/Logic and Bit Operations/Bitwise Operator  logicop=AND  UseBitMask=off  NumInputPorts=2  BitMask=bin2dec('11011001')  BitMaskRealWorld=Stored Integer
      settings: AttributesFormatString=%<logicop>
  Bitwise Operator1 : simulink/Logic and Bit Operations/Bitwise Operator  logicop=AND  UseBitMask=off  NumInputPorts=2  BitMask=bin2dec('11011001')  BitMaskRealWorld=Stored Integer
  Constant : Constant  Value=0
  Constant1 : Constant  OutDataTypeStr=uint8
  CopyRight2 : Subsystem  Description=|  mask(Copyright Information){none=on}
      | Copyright info block.                                               
      |                                                                     
      | Place copyright information at the top of every subsystem in design.
      mask prompts: none "No parameters"
      mask help: Place copyright information at the top of every subsystem in design.
      mask Display:
      | NxtrConf = 'Nexteer Confidential';
      | 
      | sys = bdroot; %handle for the current model ("system")
      | first = get_param(sys,'Created');
      | first = first(end-3:end);  %year is last four digits
      | 
      | last = get_param(sys,'LastModifiedDate');
      | if isempty(last)
      |     last = datestr(now,'yyyy');
      | else
      |     last = last(end-3:end);
      | end
      | 
      | if strcmp(first,last)
      |     fprintf('%s -- Copyright %s Nexteer',NxtrConf,first)
      | else
      |     fprintf('%s -- %s%s- %s Nexteer',NxtrConf,char(169),first,last)
      | end
  Data Store Read1 : DataStoreRead  DataStoreName=SciRxIdx
  Data Store Read2 : DataStoreRead  DataStoreName=SciRxProcIdx
  Data Store Read3 : DataStoreRead  DataStoreName=SciRxIdxMax
  Data Store Read4 : DataStoreRead  DataStoreName=SciRxSetBreakLoop
  Data Store Read5 : DataStoreRead  DataStoreName=SciGlbRxBuf
  Data Store Read6 : DataStoreRead  DataStoreName=SciRxIdx
  Data Store Write : DataStoreWrite  DataStoreName=SciRxIdx
  IMCARBN_PATIDMASKVAL_CNT_U08 : Constant  Value=224  OutDataTypeStr=uint8
  IMCARBN_PATIDN_CNT_U08 : Constant  Value=160  OutDataTypeStr=uint8
  If : If  NumInputs=2  IfExpression=u1 == u2
      settings: AttributesFormatString=%<IfExpression>
  If Action Subsystem : Subsystem  TreatAsAtomicUnit=on
  If Action Subsystem1 : Subsystem  TreatAsAtomicUnit=on
  Relational Operator : RelationalOperator  Operator=<  OutDataTypeStr=boolean
  Relational Operator1 : RelationalOperator  Operator===  OutDataTypeStr=boolean
  RollovrAdd : Subsystem
  Selector : Selector  IndexMode=Zero-based  InputPortWidth=8  IndexOptions=Index vector (port)  Indices=[0]  OutputSizes=1
  While Iterator : WhileIterator  MaxIters=-1  ResetStates=reset
  wires:
  Data Store Read2/1 -> Selector/2
  Selector/1 -> Bitwise Operator/1
  If/2 -> If Action Subsystem1/Action
  If/1 -> If Action Subsystem/Action
  IMCARBN_PATIDMASKVAL_CNT_U08/1 -> Bitwise Operator/2
  Bitwise Operator/1 -> If/1
  Bitwise Operator1/1 -> While Iterator/1
  IC/1 -> While Iterator/2
  Data Store Read1/1 -> Relational Operator/1
  Data Store Read3/1 -> Relational Operator/2
  Data Store Read4/1 -> Relational Operator1/1
  Constant/1 -> Relational Operator1/2
  Relational Operator/1 -> Bitwise Operator1/1
  Relational Operator1/1 -> Bitwise Operator1/2
  IMCARBN_PATIDN_CNT_U08/1 -> If/2
  Data Store Read5/1 -> Selector/1
  Data Store Read6/1 -> RollovrAdd/1(In1)
  Constant1/1 -> RollovrAdd/2(In2)
  RollovrAdd/1(Out1) -> Data Store Write/1

== system CM745A_Sci30CfgAndUse/Sci30CfgAndUse/Sci30CfgAndUsePer1/Update DTS registers/CopyRight2 ==

== system CM745A_Sci30CfgAndUse/Sci30CfgAndUse/Sci30CfgAndUsePer1/Update DTS registers/If Action Subsystem1 ==
  Action Port : ActionPort  ActionType=then
  Add1 : Sum  OutDataTypeStr=Inherit: Inherit via back propagation
  Constant4 : Constant  OutDataTypeStr=uint8
  CopyRight2 : Subsystem  Description=|  mask(Copyright Information){none=on}
      | Copyright info block.                                               
      |                                                                     
      | Place copyright information at the top of every subsystem in design.
      mask prompts: none "No parameters"
      mask help: Place copyright information at the top of every subsystem in design.
      mask Display:
      | NxtrConf = 'Nexteer Confidential';
      | 
      | sys = bdroot; %handle for the current model ("system")
      | first = get_param(sys,'Created');
      | first = first(end-3:end);  %year is last four digits
      | 
      | last = get_param(sys,'LastModifiedDate');
      | if isempty(last)
      |     last = datestr(now,'yyyy');
      | else
      |     last = last(end-3:end);
      | end
      | 
      | if strcmp(first,last)
      |     fprintf('%s -- Copyright %s Nexteer',NxtrConf,first)
      | else
      |     fprintf('%s -- %s%s- %s Nexteer',NxtrConf,char(169),first,last)
      | end
  Data Store Read5 : DataStoreRead  DataStoreName=SciDiagcRxMaxDataErrCntr
  Data Store Write3 : DataStoreWrite  DataStoreName=SciDiagcRxMaxDataErrCntr
  wires:
  Data Store Read5/1 -> Add1/1
  Add1/1 -> Data Store Write3/1
  Constant4/1 -> Add1/2
